simulink model "sipro_B35_diffSolvers"  (R2018a)
settings: Solver=VariableStepAuto  StartTime=0.0  StopTime=10.0  FixedStep=ts  RelTol=1e-3
values from neighbouring files (symbols this model uses):
  C = [1, 0]    [main.m]
  D = 0    [main.m]
  den = [1 0 4]    [main.m]
  KD = 0.75    [main.m]
  KI = 2.70    (= 2.7)    [main.m]
  KP = 1.25    [main.m]
  num = [w0*w0*G]    [main.m]
  ts = 0.05    [main.m]
undefined symbols (not defined in the file or in its folder): atilde, btilde
libraries: simulink x1
settings Model: Creator=Sampreet Sarkar  LastModifiedBy=Sampreet Sarkar

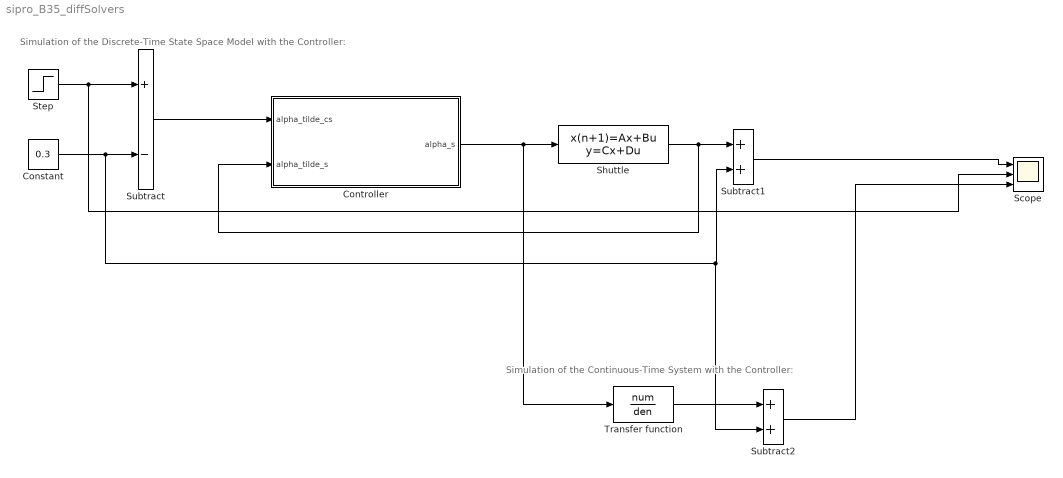
== system sipro_B35_diffSolvers ==
  note: Simulation of the Discrete-Time State Space Model with the Controller:
  note: Simulation of the Continuous-Time System with the Controller:
  Constant : Constant  Value=0.3
  Controller : Subsystem
  Scope : Scope  NumInputPorts=3
  "Shuttle " : DiscreteStateSpace  A=atilde  B=btilde  C=C  D=D  SampleTime=ts
  Step : Step  Before=0.3  After=0.27  SampleTime=ts
  Subtract : Sum  Inputs=+-
  Subtract1 : Sum
  Subtract2 : Sum
  "Transfer function " : TransferFcn  Numerator=num  Denominator=den
  wires:
  Subtract/1 -> Controller/1(alpha_tilde_cs)
  Constant/1 -> Subtract2/2, Subtract1/2, Subtract/2
  "Shuttle "/1 -> Controller/2(alpha_tilde_s), Subtract1/1
  Subtract1/1 -> Scope/1
  Step/1 -> Scope/2, Subtract/1
  "Transfer function "/1 -> Subtract2/1
  Controller/1(alpha_s) -> "Transfer function "/1, "Shuttle "/1
  Subtract2/1 -> Scope/3

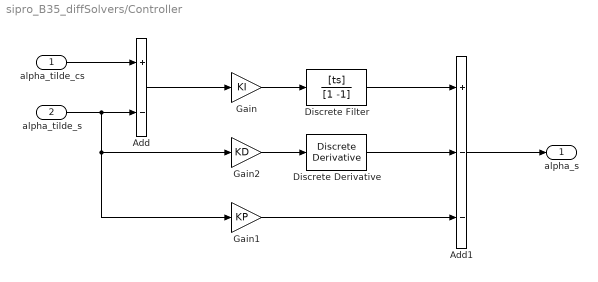
== system sipro_B35_diffSolvers/Controller ==
  alpha_tilde_cs : Inport
  alpha_tilde_s : Inport  Port=2
  Add : Sum  Inputs=+-
  Add1 : Sum  Inputs=+--
  Discrete Derivative : simulink/Discrete/Discrete Derivative  gainval=1.0  ICPrevScaledInput=0.0  OutMin=[]  OutMax=[]  OutDataType=fixdt(1, 16)  OutScaling=2^-10  DoSatur=off
  Discrete Filter : DiscreteFilter  Numerator=[ts]  Denominator=[1 -1]
  Gain : Gain  Gain=KI
  Gain1 : Gain  Gain=KP
  Gain2 : Gain  Gain=KD
  alpha_s : Outport
  wires:
  Gain2/1 -> Discrete Derivative/1
  Discrete Filter/1 -> Add1/1
  Add/1 -> Gain/1
  Gain/1 -> Discrete Filter/1
  alpha_tilde_s/1 -> Gain1/1, Gain2/1, Add/2
  Discrete Derivative/1 -> Add1/2
  alpha_tilde_cs/1 -> Add/1
  Gain1/1 -> Add1/3
  Add1/1 -> alpha_s/1
